simulink model "PID_analog"  (R2015a)
settings: Solver=ode45  StartTime=0.0  StopTime=10  RelTol=1e-3
libraries: fl_lib x21, nesl_utility x3
settings Model: Creator=ahmed alaa  LastModifiedBy=ahmed alaa

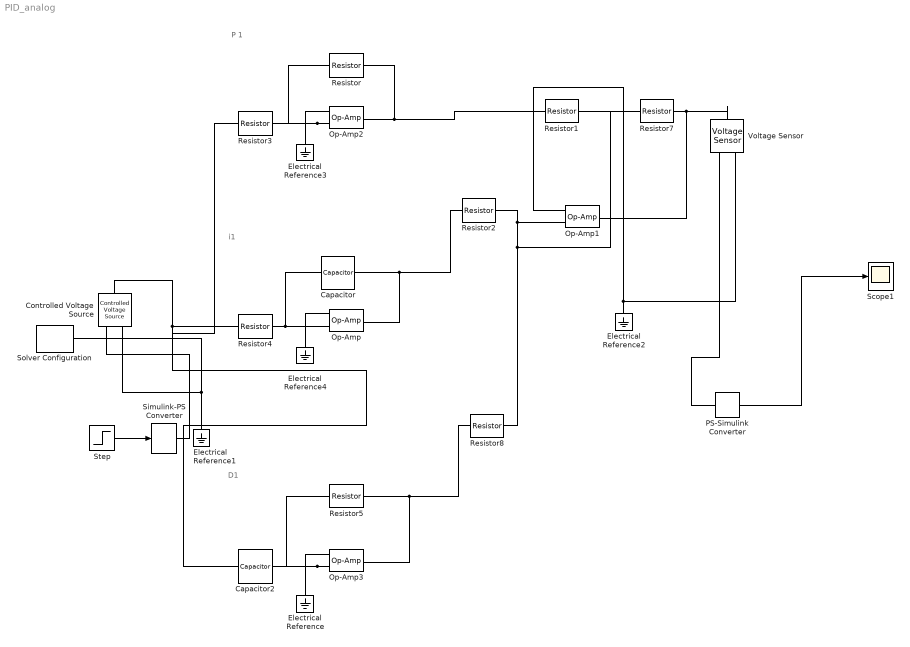
== system PID_analog ==
  note: D1
  note: i1
  note: P
      | 1
  Capacitor : fl_lib/Electrical/Electrical Elements/Capacitor  c=1e-6 F  r=1e-6 Ohm  g=0 1/Ohm  i_specify=off  i_priority=High  i=0 A  v_specify=off  v_priority=High  v=0 V  vc_specify=off  vc_priority=High  vc=0 V
  Capacitor2 : fl_lib/Electrical/Electrical Elements/Capacitor  c=1e-6 F  r=1e-6 Ohm  g=0 1/Ohm  i_specify=off  i_priority=High  i=0 A  v_specify=off  v_priority=High  v=0 V  vc_specify=off  vc_priority=High  vc=0 V
  Controlled Voltage Source : fl_lib/Electrical/Electrical Sources/Controlled Voltage Source
  Electrical Reference{,1..4} (5 alike) : fl_lib/Electrical/Electrical Elements/Electrical Reference
  Op-Amp{,1..3} (4 alike) : fl_lib/Electrical/Electrical Elements/Op-Amp  outI_specify=off  outI_priority=High  outI=0 A
  PS-Simulink Converter : nesl_utility/PS-Simulink Converter  PhysicalDomain=network_engine_domain  SubClassName=ps_output  LeftPortType=input  RightPortType=output  PseudoPeriodic=off  Frequencies=[]  Unit=1  AffineConversion=off
  Resistor{,1..5,7..8} (8 alike) : fl_lib/Electrical/Electrical Elements/Resistor  R=1 Ohm  i_specify=off  i_priority=High  i=0 A  v_specify=off  v_priority=High  v=0 V
  Scope1 : Scope
  Simulink-PS Converter : nesl_utility/Simulink-PS Converter  PhysicalDomain=network_engine_domain  SubClassName=ps_input  LeftPortType=input  RightPortType=output  PseudoPeriodic=off  Frequencies=[]  NoiseDistribution=none  NoiseParameters=[]  Unit=1  AffineConversion=off  InputFiltering=off  SimscapeFilterOrder=1  InputFilterTimeConstant=0.001  UdotUserProvided=1
  Solver Configuration : nesl_utility/Solver Configuration  PhysicalDomain=network_engine_domain  SubClassName=solver  LeftPortType=input  RightPortType=generic  Accelerate=off  Tones=[]  Harmonics=[]  SimulateNoise=off  Profile=off  UseLocalSampling=off  EnableSwitchedLinearOptims=on  FrequencyDomain=off  UseCCode=off  RelTol=0.001  AbsTol=1e-06  MinStep=1e-09  ToWorkspace=off  RevertToSquareIcSolve=off  NumHomotopyIterations=100  DoDC=off  ResidualTolerance=1e-09  UseLocalSolver=off  LocalSolverChoice=NE_BACKWARD_EULER_ADVANCER  LocalSolverSampleTime=0.001  DoFixedCost=off  MaxNonlinIter=3  MaxModeIter=2  LinearAlgebra=Sparse  DelaysMemoryBudget=1024  AutomaticFiltering=on  FilteringTimeConstant=0.001
  Step : Step  SampleTime=0
  Voltage Sensor : fl_lib/Electrical/Electrical Sensors/Voltage Sensor
  wires:
  PS-Simulink Converter/1 -> Scope1/1
  Step/1 -> Simulink-PS Converter/1
  connections:
  Resistor2/RConn1 -- Resistor1/RConn1 -- Resistor7/LConn1 -- Resistor8/RConn1 -- Op-Amp1/LConn2
  Resistor7/RConn1 -- Op-Amp1/RConn1 -- Voltage Sensor/LConn1
  Op-Amp1/LConn1 -- Voltage Sensor/RConn2 -- Electrical Reference2/LConn1
  Electrical Reference1/LConn1 -- Solver Configuration/RConn1 -- Controlled Voltage Source/RConn2
  Controlled Voltage Source/RConn1 -- Simulink-PS Converter/RConn1
  Voltage Sensor/RConn1 -- PS-Simulink Converter/LConn1
  Op-Amp2/LConn2 -- Resistor3/RConn1 -- Resistor/LConn1
  Op-Amp2/LConn1 -- Electrical Reference3/LConn1
  Resistor/RConn1 -- Resistor1/LConn1 -- Op-Amp2/RConn1
  Electrical Reference4/LConn1 -- Op-Amp/LConn1
  Controlled Voltage Source/LConn1 -- Capacitor2/LConn1 -- Resistor3/LConn1 -- Resistor4/LConn1
  Resistor4/RConn1 -- Op-Amp/LConn2 -- Capacitor/LConn1
  Op-Amp/RConn1 -- Resistor2/LConn1 -- Capacitor/RConn1
  Op-Amp3/LConn2 -- Capacitor2/RConn1 -- Resistor5/LConn1
  Resistor5/RConn1 -- Resistor8/LConn1 -- Op-Amp3/RConn1
  Op-Amp3/LConn1 -- Electrical Reference/LConn1
